simulink model "lab2"  (R2015b)
settings: Solver=FixedStepAuto  StartTime=0  StopTime=0.0015  FixedStep=Ts  RelTol=1e-3
values from neighbouring files (symbols this model uses):
  A = 1    [dev_digicomm_lab2.m]
  N1 = 0.1    [dev_digicomm_lab2.m]
  N2 = 0.2    [dev_digicomm_lab2.m]
  N3 = 0.25    [dev_digicomm_lab2.m]
libraries: simulink x2
settings Model: Creator=Devin  LastModifiedBy=trejo
settings DataIOCC: SaveFormat=Array
settings HardwareCC: ProdBitPerPointer=32  ProdLargestAtomicFloat=None  ProdIntDivRoundTo=Undefined  ProdEndianess=Unspecified  ProdWordSize=32  ProdHWDeviceType=32-bit Generic
settings GRTTargetCC: GeneratePreprocessorConditionals=Disable all
settings ConfigComp: CovModelRefEnable=Off

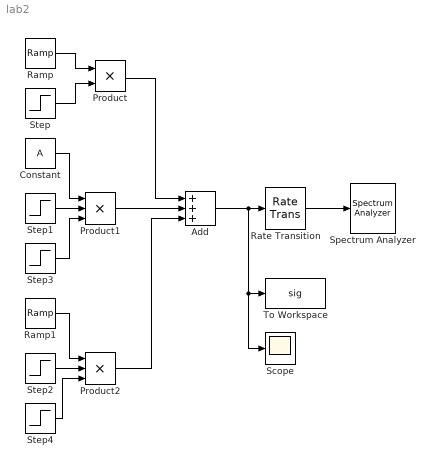
== system lab2 ==
  Add : Sum  Inputs=+++
  Constant : Constant  Value=A
  Product : Product
  Product1 : Product  Inputs=3
  Product2 : Product  Inputs=3
  Ramp : simulink/Sources/Ramp  slope=A/N1  start=0  X0=0
  Ramp1 : simulink/Sources/Ramp  slope=-A/(N3)  start=N1+N2  X0=A
  Rate Transition : RateTransition  OutPortSampleTimeOpt=Inherit  OutPortSampleTime=Ts
  Scope : Scope
  Spectrum Analyzer : SpectrumAnalyzer
  Step : Step  Time=N1  Before=1  After=0  SampleTime=0
  Step1 : Step  Time=N1  SampleTime=0
  Step2 : Step  Time=N1+N2  SampleTime=0
  Step3 : Step  Time=N1+N2  Before=1  After=0  SampleTime=0
  Step4 : Step  Time=N1+N2+N3  Before=1  After=0  SampleTime=0
  To Workspace : ToWorkspace  VariableName=sig  SaveFormat=Timeseries  SampleTime=-1
  wires:
  Step/1 -> Product/2
  Ramp/1 -> Product/1
  Constant/1 -> Product1/1
  Step1/1 -> Product1/2
  Ramp1/1 -> Product2/1
  Step2/1 -> Product2/2
  Product/1 -> Add/1
  Product1/1 -> Add/2
  Product2/1 -> Add/3
  Add/1 -> Rate Transition/1, To Workspace/1, Scope/1
  Step3/1 -> Product1/3
  Step4/1 -> Product2/3
  Rate Transition/1 -> Spectrum Analyzer/1
